simulink model "flythedrone"  (R2019b)
settings: Solver=FixedStepAuto  StartTime=0.0  StopTime=100  RelTol=1e-3
InitFcn:
  | load('BusDefinitions.mat')
values from neighbouring files (symbols this model uses):
  A1_kalman = eval(subs(A1_sampled, t))    [simulation_matlab.m]
  A2_kalman = eval(subs(A2_sampled, t))    [simulation_matlab.m]
  A_s_double = eval(subs(Ad_double,Ts))    [simulation_matlab.m]
  A_s_single = eval(subs(Ad_single,Ts))    [simulation_matlab.m]
  B1_kalman = eval(subs(B1_sampled, t))    [simulation_matlab.m]
  B2_kalman = eval(subs(B2_sampled, t))    [simulation_matlab.m]
  B_s_double = eval(subs(Bd_double,Ts))    [simulation_matlab.m]
  B_s_single = eval(subs(Bd_single,Ts))    [simulation_matlab.m]
  C1_kalman = C1_sampled    [simulation_matlab.m]
  C2_kalman = C2_sampled    [simulation_matlab.m]
  C_double = [1 0]    [simulation_matlab.m]
  C_single = [1]    [simulation_matlab.m]
  D1_kalman = D1_sampled    [simulation_matlab.m]
  D2_kalman = D2_sampled    [simulation_matlab.m]
  D_double = [0]    [simulation_matlab.m]
  D_single = [0]    [simulation_matlab.m]
  Kaileron = lqr(Aaileron, Baileron, Qaileron, Raileron)    [simulation_matlab.m]
  Kelevator = lqr(Aelevator, Belevator, Qelevator, Relevator)    [simulation_matlab.m]
  Krudder = lqr(Arudder, Brudder, Qrudder, Rrudder)    [simulation_matlab.m]
  Kthrust = lqr(Athrust, Bthrust, Qthrust, Rthrust)    [simulation_matlab.m]
  M_motor = [1, 1, 1, -1;             1, 1, -1, 1;             1, -1, -1, -1;             1, -1, 1, 1 ]    [simulation_matlab.m]
  omega_c = 2*pi *20    (= 125.663706144)    [simulation_matlab.m]
  q1_noise = 1    [simulation_matlab.m]
  q2_noise = 1    [simulation_matlab.m]
  q3_noise = 1    [simulation_matlab.m]
  q4_noise = 1    [simulation_matlab.m]
  q5_noise = 1    [simulation_matlab.m]
  q_single = cov(out.In_Out_Data{1}.Values.Data)*10000000000000    [simulation_matlab.m]
  r1_noise = 100    [simulation_matlab.m]
  r2_noise = 100    [simulation_matlab.m]
  r3_noise = 100    [simulation_matlab.m]
  r4_noise = 100    [simulation_matlab.m]
  r5_noise = 100    [simulation_matlab.m]
  r_single = cov(out.In_Out_Data{2}.Values.Data)    [simulation_matlab.m]
  Ts = 0.005    [simulation_matlab.m]
undefined symbols (not defined in the file or in its folder): codertarget, DiscIntNeverNeededParam, Discrete, Time
libraries: ctrlSharedLib x12, simulink x1
settings Model: ExtModeTrigDuration=80  Creator=Sankalp Bhan  LastModifiedBy=cwhipp
settings OptimizationCC: PassReuseOutputArgsThreshold=0  MaxStackSize=64
settings DebuggingCC: ParameterTunabilityLossMsg=error  ArithmeticOperatorsInVariantConditions=warning
settings HardwareCC: ProdBitPerPointer=32  ProdBitPerSizeT=32  ProdBitPerPtrDiffT=32  ProdLargestAtomicInteger=Long  ProdWordSize=32  ProdHWDeviceType=ARM Compatible->ARM 9  UseEmbeddedCoderFeatures=off
settings SFSimCC: SimUseLocalCustomCode=off  MATLABDynamicMemAlloc=off
settings RTWCC: SystemTargetFile=ert.tlc  HardwareBoard=PARROT Mambo  TLCOptions="-aInlineSetEventsForThisBaseRateFcn=TLC_FALSE -aSuppressMultiTaskScheduler=TLC_FALSE   -aRateBasedStepFcn=1"  TemplateMakefile=ert_default_tmf  GenerateReport=on  RTWUseLocalCustomCode=off  Toolchain=Sourcery G++ Lite GNU Toolchain for Drones  LaunchReport=on
settings CodeAppCC: ForceParamTrailComments=on  OperatorAnnotations=on  StateflowObjectComments=on
settings ERTTargetCC: ERTCustomFileBanners=off  MatFileLogging=on  SupportContinuousTime=on  SupportNonInlinedSFcns=on  RemoveResetFunc=off  ModelStepFunctionPrototypeControlCompliant=off

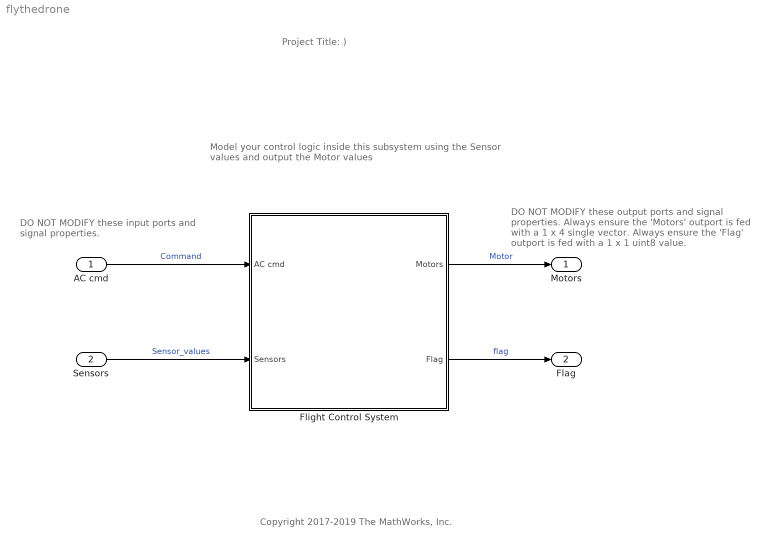
== system flythedrone ==
  note: Model your control logic inside this subsystem
      | using the Sensor values and output the
      | Motor values
  note: DO NOT MODIFY these output ports
      | and signal properties.
      |
      |
      |
      | Always ensure the 'Motors' outport
      | is fed with a 1 x 4 single vector.
      |
      |
      |
      |
      |
      | Always ensure the 'Flag' outport is
      | fed with a 1 x 1 uint8 value.
  note: DO NOT MODIFY these input
      | ports and signal properties.
  note: Copyright 2017-2019 The MathWorks, Inc.
  note: Project Title: )
  AC cmd : Inport  OutDataTypeStr=Bus: CommandBus  BusOutputAsStruct=on
  Sensors : Inport  Port=2  OutDataTypeStr=Bus: SensorsBus  BusOutputAsStruct=on
  Flight Control System : Subsystem  InitFcn=codertarget.parrot.internal.fcsSubsystemCallback(gcb);
  Motors : Outport  OutDataTypeStr=single  PortDimensions=[1 4]  VectorParamsAs1DForOutWhenUnconnected=off
  Flag : Outport  Port=2  OutDataTypeStr=uint8  PortDimensions=1  VectorParamsAs1DForOutWhenUnconnected=off
  wires:
  Flight Control System/1(Motors) -> Motors/1  "Motor"
  AC cmd/1 -> Flight Control System/1(AC cmd)  "Command"
  Sensors/1 -> Flight Control System/2(Sensors)  "Sensor_values"
  Flight Control System/2(Flag) -> Flag/1  "flag"

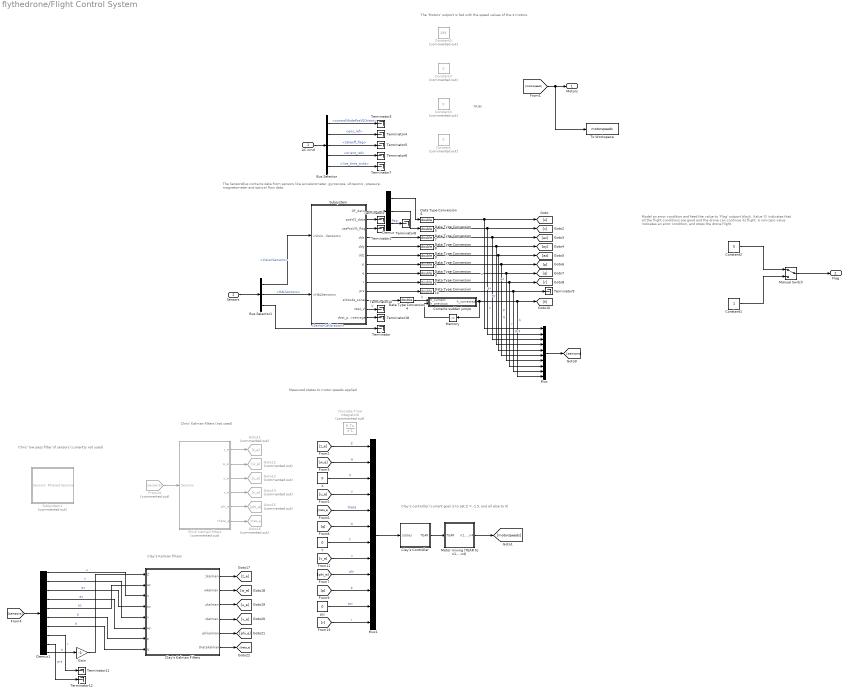
== system flythedrone/Flight Control System ==
  note: Measured states to motor speeds applied
  note: TRIM
  note: The 'Motors' outport is fed with the speed values of the 4 motors.
  note: Model an error condition and feed the value to 'Flag' outport block.
      | Value '0' indicates that all the flight conditions are good and the drone
      | can continue its flight.
      | A non-zero value indicates an error condition, and stops the drone
      | flight.
  note: The SensorsBus contains data from sensors like
      | accelerometer, gyroscope, ultrasonic, pressure,
      | magnetometer and optical flow data.
  note: Chris' Kalman filters (not used)
  note: Chris' low pass filter of sensors
      | (currently not used)
  note: Clay's Kalman filters
  note: Clay's controller (current goal is to set Z = -1.5, and all else to 0)
  AC cmd : Inport
  Sensors : Inport  Port=2
  Bus Selector : BusSelector  OutputSignals=controlModePosVSOrient,pos_ref,takeoff_flag,orient_ref,live_time_ticks
  Bus Selector1 : BusSelector  OutputSignals=VisionSensors,HALSensors,SensorCalibration
  Chris' kalman filters : Subsystem  Commented=on
  Clay's Controller : Subsystem
  Clay's Kalman Filters : Subsystem
  Constant : Constant  Commented=on  Value=0  SampleTime=Ts
  Constant1 : Constant  OutDataTypeStr=uint8
  Constant2 : Constant  Value=0  OutDataTypeStr=uint8
  Constant3 : Constant  Commented=on  Value=0  SampleTime=Ts
  Constant4 : Constant  Commented=on  Value=0  SampleTime=Ts
  Constant5 : Constant  Commented=on  Value=293  SampleTime=Ts
  Corrects sudden jumps : MATLAB Function  TreatAsAtomicUnit=on
  Data Type Conversion{1..10} (10 alike) : DataTypeConversion  OutDataTypeStr=double
  Demux : Demux  Outputs=3
  Demux1 : Demux  Outputs=10
  Discrete-Time Integrator6 : DiscreteIntegrator  Commented=on  SampleTime=-1  ICPrevOutput=DiscIntNeverNeededParam  ICPrevScaledInput=DiscIntNeverNeededParam
  From14 : From  Commented=on  GotoTag=sensors
  Gain : Gain  Gain=-1
  Goto11 : Goto  Commented=on  GotoTag=z_e
  Goto12 : Goto  Commented=on  GotoTag=w_e
  Goto13 : Goto  Commented=on  GotoTag=u_e
  Goto14 : Goto  Commented=on  GotoTag=v_e
  Goto15 : Goto  Commented=on  GotoTag=phi_e
  Goto16 : Goto  Commented=on  GotoTag=theta_e
  Manual Switch : ManualSwitch
  Memory : Memory
  Motor mixing (TEAR to n1,...,n4) : Subsystem
  Mux : Mux  Inputs=10
  Mux1 : Mux  Inputs=12
  Subsystem : Subsystem
  Subsystem1 : Subsystem  Commented=on
  Terminator{,1..12,18} (14 alike) : Terminator
  To Workspace : ToWorkspace  VariableName=motorspeeds  SaveFormat=Structure With Time  SampleTime=-1
  X : Constant  Value=0  SampleTime=0.005
  Y : Constant  Value=0  SampleTime=0.005
  psi : Constant  Value=0  SampleTime=0.005
  Motors : Outport  VectorParamsAs1DForOutWhenUnconnected=off
  Flag : Outport  Port=2  VectorParamsAs1DForOutWhenUnconnected=off
  wires:
  AC cmd/1 -> Bus Selector/1
  Sensors/1 -> Bus Selector1/1
  Bus Selector/1 -> Terminator3/1  "<controlModePosVSOrient>"
  Bus Selector/2 -> Terminator4/1  "<pos_ref>"
  Bus Selector/3 -> Terminator5/1  "<takeoff_flag>"
  Bus Selector/4 -> Terminator6/1  "<orient_ref>"
  Bus Selector/5 -> Terminator7/1  "<live_time_ticks>"
  Manual Switch/1 -> Flag/1
  Constant2/1 -> Manual Switch/1
  Constant1/1 -> Manual Switch/2
  [motorspeeds] -> To Workspace/1, Motors/1
  Bus Selector1/1 -> Subsystem/1(<VisionSensors>)  "<VisionSensors>"
  Bus Selector1/2 -> Subsystem/2(<HALSensors>)  "<HALSensors>"
  Bus Selector1/3 -> Terminator/1  "<SensorCalibration>"
  Subsystem/1(OF_data) -> Demux/1
  Subsystem/4(ddx) -> Data Type Conversion7/1
  Subsystem/5(ddy) -> Data Type Conversion8/1
  Subsystem/6(ddz) -> Data Type Conversion9/1
  Subsystem/7(p) -> Data Type Conversion2/1
  Subsystem/9(r) -> Data Type Conversion1/1
  Subsystem/11(altitude_sonar) -> Data Type Conversion4/1
  Subsystem/13(vbat_percentage) -> Terminator18/1
  Subsystem/8(q) -> Data Type Conversion3/1
  Subsystem/3(usePosVIS_flag) -> Terminator1/1
  Subsystem/2(posVIS_data) -> Terminator2/1
  Demux/1 -> Data Type Conversion6/1
  Demux/2 -> Data Type Conversion5/1
  Demux/3 -> Terminator8/1  "flag"
  Subsystem/10(prs) -> Data Type Conversion10/1
  Data Type Conversion1/1 -> Mux/8, [r]  "r"
  Data Type Conversion2/1 -> Mux/6, [p]  "p"
  Data Type Conversion3/1 -> Mux/7, [q]  "q"
  Data Type Conversion5/1 -> Mux/2, [v]  "v"
  Data Type Conversion6/1 -> [u], Mux/1  "u"
  Data Type Conversion7/1 -> Mux/3, [ax]  "ax"
  Data Type Conversion8/1 -> Mux/4, [ay]  "ay"
  Data Type Conversion9/1 -> Mux/5, [az]  "az"
  Data Type Conversion10/1 -> Mux/9, Terminator9/1  "prs"
  Subsystem/12(vbat_V) -> Terminator10/1  "V"
  Mux1/1 -> Clay's Controller/1(states)
  Motor mixing (TEAR to n1,...,n4)/1(n1,...,n4) -> [motorspeeds]
  [z_e] -> Mux1/1  "Z"
  [w_e] -> Mux1/2  "w"
  [u_e] -> Mux1/4  "u"
  [theta_e] -> Mux1/5  "theta"
  [q] -> Mux1/6  "q"
  Y/1 -> Mux1/7  "Y"
  [p] -> Mux1/10  "p"
  [phi_e] -> Mux1/9  "phi"
  [v_e] -> Mux1/8  "v"
  psi/1 -> Mux1/11  "psi"
  [r] -> Mux1/12  "r"
  Clay's Controller/1(TEAR) -> Motor mixing (TEAR to n1,...,n4)/1(TEAR)
  Mux/1 -> [sensors]
  From14/1 -> Chris' kalman filters/1(Sensors)
  Chris' kalman filters/1(z_e) -> Goto11/1
  Chris' kalman filters/2(w_e) -> Goto12/1
  Chris' kalman filters/3(u_e) -> Goto13/1
  Chris' kalman filters/4(v_e) -> Goto14/1
  Chris' kalman filters/5(phi_e) -> Goto15/1
  Chris' kalman filters/6(theta_e) -> Goto16/1
  X/1 -> Mux1/3  "X"
  Data Type Conversion4/1 -> Corrects sudden jumps/1(h_current)  "h"
  Corrects sudden jumps/1(h_corrected) -> [h], Mux/10, Memory/1  "h"
  Memory/1 -> Corrects sudden jumps/2(h_previous)
  Clay's Kalman Filters/6(thetakalman) -> [theta_e]
  Clay's Kalman Filters/1(zkalman) -> [z_e]
  Clay's Kalman Filters/5(phikalman) -> [phi_e]
  Clay's Kalman Filters/2(wkalman) -> [w_e]
  Clay's Kalman Filters/3(ukalman) -> [u_e]
  Clay's Kalman Filters/4(vkalman) -> [v_e]
  [sensors] -> Demux1/1
  Demux1/1 -> Clay's Kalman Filters/3(u)  "u"
  Demux1/2 -> Clay's Kalman Filters/5(v)  "v"
  Demux1/3 -> Clay's Kalman Filters/4(ax)  "ax"
  Demux1/4 -> Clay's Kalman Filters/6(ay)  "ay"
  Demux1/5 -> Clay's Kalman Filters/2(az)  "az"
  Demux1/6 -> Clay's Kalman Filters/7(p)  "p"
  Demux1/7 -> Clay's Kalman Filters/8(q)  "q"
  Demux1/8 -> Terminator11/1  "r"
  Gain/1 -> Clay's Kalman Filters/1(Z)
  Demux1/10 -> Gain/1  "h"
  Demux1/9 -> Terminator12/1  "prs"

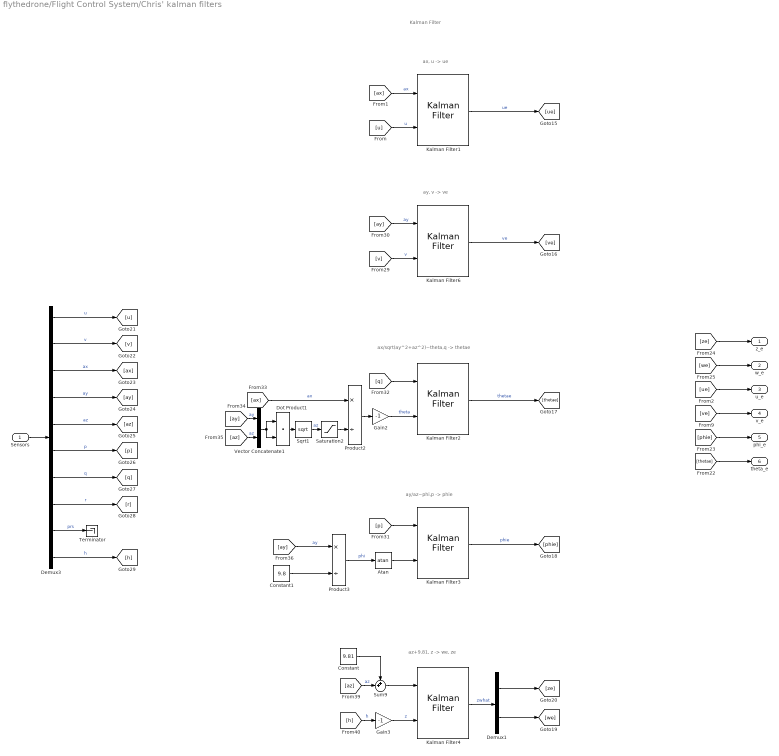
== system flythedrone/Flight Control System/Chris' kalman filters ==
  note: Kalman Filter
  note: ay, v -> ve
  note: ax, u -> ue
  note: ax/sqrt(ay^2+az^2)~theta,q -> thetae
  note: ay/az~phi,p -> phie
  note: az+9.81, z -> we, ze
  Sensors : Inport
  Atan : Trigonometry  Operator=atan
  Constant : Constant  Value=9.81
  Constant1 : Constant  Value=9.8
  Demux1 : Demux  Outputs=2
  Demux3 : Demux  Outputs=10
  Dot Product1 : DotProduct  OutMin=0.0001  InputSameDT=on  OutDataTypeStr=Inherit: Inherit via internal rule
  Gain2 : Gain  Gain=-1
  Gain3 : Gain  Gain=-1
  Kalman Filter{1..3,6} (4 alike) : ctrlSharedLib/Kalman Filter  TimeDomain=Discrete-Time  UseCurrentEstimator=on  ModelSource=Individual A, B, C, D matrices  ModelSourceVariable=ss(0.95,1,1,0,1)  A=A_s_single  B=B_s_single  C=C_single  D=D_single  NumberOfStates=1  NumberOfInputs=1  NumberOfOutputs=1  InitialEstimateSource=Dialog  X0=[0]  P0=10  UseK=off  UseGH=off  NumberOfProcessNoiseInputs=1  G=1  TimeInvariantG=on  H=0  TimeInvariantH=on  Q=[1]*q_single  TimeInvariantQ=on  R=[1]*r_single*10000  TimeInvariantR=on  N=0  TimeInvariantN=on  AddInputPort=on  AddEnablePort=off  OutputEstimatedY=off  OutputP=off  Ts=Ts
      settings: SourceProductBaseCode=CT
  Kalman Filter4 : ctrlSharedLib/Kalman Filter  TimeDomain=Discrete-Time  UseCurrentEstimator=on  ModelSource=Individual A, B, C, D matrices  ModelSourceVariable=ss(0.95,1,1,0,1)  A=A_s_double  B=B_s_double  C=C_double  D=D_double  NumberOfStates=1  NumberOfInputs=1  NumberOfOutputs=1  InitialEstimateSource=Dialog  X0=[0]  P0=10  UseK=off  UseGH=off  NumberOfProcessNoiseInputs=1  G=1  TimeInvariantG=on  H=0  TimeInvariantH=on  Q=[0 0; 0 1]*q_single  TimeInvariantQ=on  R=[1]*r_single*10000  TimeInvariantR=on  N=0  TimeInvariantN=on  AddInputPort=on  AddEnablePort=off  OutputEstimatedY=off  OutputP=off  Ts=Ts
      settings: SourceProductBaseCode=CT
  Product2 : Product  Inputs=*/
  Product3 : Product  Inputs=*/
  Saturation2 : Saturate  UpperLimit=inf  LowerLimit=0.001
  Sqrt1 : Sqrt  SaturateOnIntegerOverflow=on
  Sum9 : Sum  Inputs=++|
  Terminator : Terminator
  Vector Concatenate1 : Concatenate
  z_e : Outport
  w_e : Outport  Port=2
  u_e : Outport  Port=3
  v_e : Outport  Port=4
  phi_e : Outport  Port=5
  theta_e : Outport  Port=6
  wires:
  [h] -> Gain3/1  "h"
  Kalman Filter1/1 -> [ue]  "ue"
  Kalman Filter6/1 -> [ve]  "ve"
  Kalman Filter2/1 -> [thetae]  "thetae"
  Kalman Filter3/1 -> [phie]  "phie"
  Demux1/2 -> [we]
  Demux1/1 -> [ze]
  Gain3/1 -> Kalman Filter4/2  "z"
  Kalman Filter4/1 -> Demux1/1  "zwhat"
  [ay] -> Product3/1  "ay"
  Product3/1 -> Atan/1  "phi"
  [p] -> Kalman Filter3/1
  [ay] -> Vector Concatenate1/1  "ay"
  [az] -> Vector Concatenate1/2  "az"
  Vector Concatenate1/1 -> Dot Product1/1, Dot Product1/2
  Dot Product1/1 -> Sqrt1/1
  [ax] -> Product2/1  "ax"
  Product2/1 -> Gain2/1
  Sqrt1/1 -> Saturation2/1  "az"
  Saturation2/1 -> Product2/2
  Gain2/1 -> Kalman Filter2/2  "theta"
  [q] -> Kalman Filter2/1
  [ay] -> Kalman Filter6/1  "ay"
  [v] -> Kalman Filter6/2  "v"
  [u] -> Kalman Filter1/2  "u"
  [ax] -> Kalman Filter1/1  "ax"
  [az] -> Sum9/2  "az"
  Sum9/1 -> Kalman Filter4/1
  Constant/1 -> Sum9/1
  Demux3/1 -> [u]  "u"
  Sensors/1 -> Demux3/1
  Demux3/6 -> [p]  "p"
  Atan/1 -> Kalman Filter3/2
  Constant1/1 -> Product3/2
  [ze] -> z_e/1
  [we] -> w_e/1
  [ve] -> v_e/1
  [ue] -> u_e/1
  [phie] -> phi_e/1
  [thetae] -> theta_e/1
  Demux3/3 -> [ax]  "ax"
  Demux3/2 -> [v]  "v"
  Demux3/7 -> [q]  "q"
  Demux3/4 -> [ay]  "ay"
  Demux3/5 -> [az]  "az"
  Demux3/10 -> [h]  "h"
  Demux3/8 -> [r]  "r"
  Demux3/9 -> Terminator/1  "prs"

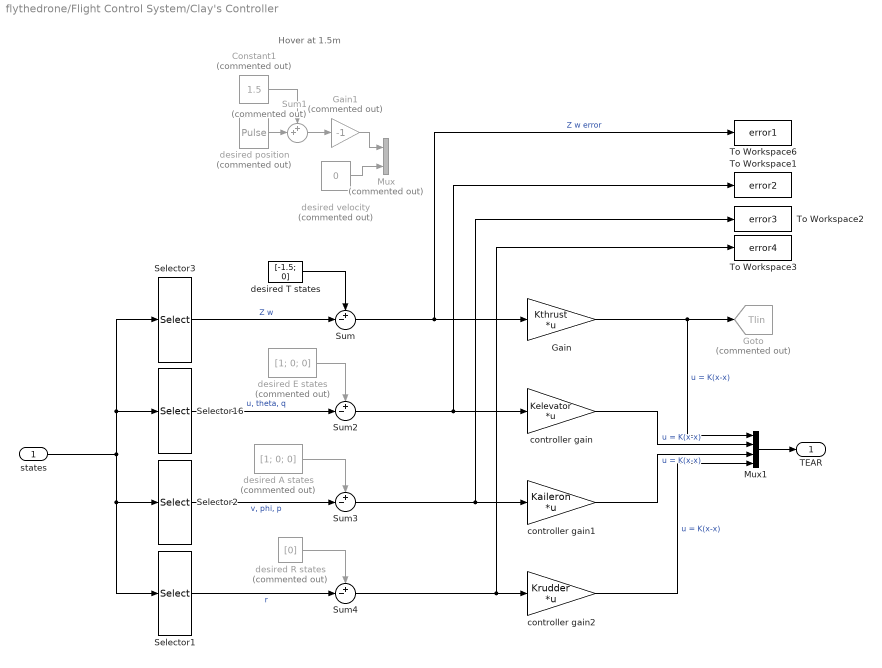
== system flythedrone/Flight Control System/Clay's Controller ==
  note: Hover at 1.5m
  states : Inport
  Constant1 : Constant  Commented=on  Value=1.5  SampleTime=0.05
  Gain : Gain  Gain=Kthrust  Multiplication=Matrix(K*u)
  Gain1 : Gain  Commented=on  Gain=-1
  Goto : Goto  Commented=on  GotoTag=Tlin  TagVisibility=global
  Mux : Mux  Commented=on  Inputs=2
  Mux1 : Mux
  Selector1 : Selector  InputPortWidth=12  IndexOptions=Index vector (dialog)  Indices=[12]  OutputSizes=1
  Selector16 : Selector  InputPortWidth=12  IndexOptions=Index vector (dialog)  Indices=[4 5 6]  OutputSizes=1
  Selector2 : Selector  InputPortWidth=12  IndexOptions=Index vector (dialog)  Indices=[8 9 10]  OutputSizes=1
  Selector3 : Selector  InputPortWidth=12  IndexOptions=Index vector (dialog)  Indices=[1 2]  OutputSizes=1
  Sum{,2..4} (4 alike) : Sum  Inputs=+-|
  Sum1 : Sum  Commented=on  Inputs=++|
  To Workspace1 : ToWorkspace  VariableName=error2  SaveFormat=Structure With Time  SampleTime=-1
  To Workspace2 : ToWorkspace  VariableName=error3  SaveFormat=Structure With Time  SampleTime=-1
  To Workspace3 : ToWorkspace  VariableName=error4  SaveFormat=Structure With Time  SampleTime=-1
  To Workspace6 : ToWorkspace  VariableName=error1  SaveFormat=Structure With Time  SampleTime=-1
  controller gain : Gain  Gain=Kelevator  Multiplication=Matrix(K*u)
  controller gain1 : Gain  Gain=Kaileron  Multiplication=Matrix(K*u)
  controller gain2 : Gain  Gain=Krudder  Multiplication=Matrix(K*u)
  desired A states : Constant  Commented=on  Value=[1; 0; 0]  SampleTime=0.005
  desired E states : Constant  Commented=on  Value=[1; 0; 0]  SampleTime=0.005
  desired R states : Constant  Commented=on  Value=[0]  SampleTime=0.005
  desired T states : Constant  Value=[-1.5; 0]  SampleTime=0.005
  desired position : DiscretePulseGenerator  Commented=on  PulseType=Time based  Amplitude=-1.5  Period=10  PulseWidth=50
  desired velocity : Constant  Commented=on  Value=0  SampleTime=0.05
  TEAR : Outport
  wires:
  states/1 -> Selector16/1, Selector3/1, Selector2/1, Selector1/1
  desired T states/1 -> Sum/1
  Sum/1 -> To Workspace6/1, Gain/1  "Z w error"
  Gain/1 -> Goto/1, Mux1/1  "u = K(x-x)"
  desired E states/1 -> Sum2/1
  Sum2/1 -> To Workspace1/1, controller gain/1
  controller gain/1 -> Mux1/2  "u = K(x-x)"
  controller gain1/1 -> Mux1/3  "u = K(x-x)"
  desired A states/1 -> Sum3/1
  controller gain2/1 -> Mux1/4  "u = K(x-x)"
  Sum4/1 -> To Workspace3/1, controller gain2/1
  desired R states/1 -> Sum4/1
  Selector3/1 -> Sum/2  "Z w"
  Selector16/1 -> Sum2/2  "u, theta, q"
  Selector2/1 -> Sum3/2  "v, phi, p"
  Selector1/1 -> Sum4/2  "r"
  Mux1/1 -> TEAR/1
  Sum1/1 -> Gain1/1
  desired position/1 -> Sum1/2
  Gain1/1 -> Mux/1
  desired velocity/1 -> Mux/2
  Constant1/1 -> Sum1/1
  Sum3/1 -> To Workspace2/1, controller gain1/1

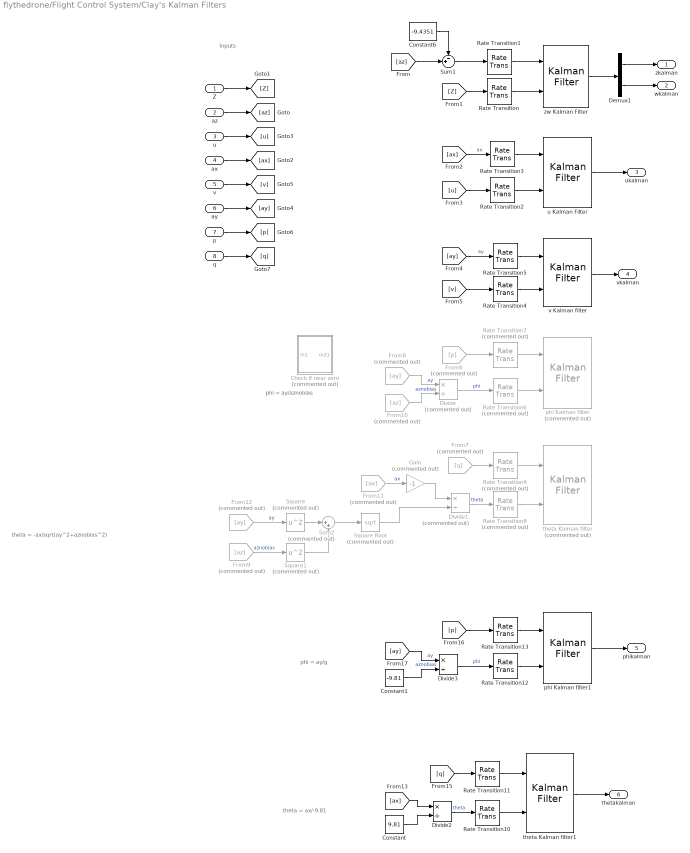
== system flythedrone/Flight Control System/Clay's Kalman Filters ==
  note: Inputs
  note: phi = ay/aznobias
  note: theta = -ax/sqrt(ay^2+aznobias^2)
  note: theta = ax/-9.81
  note: phi = ay/g
  Z : Inport
  az : Inport  Port=2
  u : Inport  Port=3
  ax : Inport  Port=4
  v : Inport  Port=5
  ay : Inport  Port=6
  p : Inport  Port=7
  q : Inport  Port=8
  Check if near zero : Subsystem  Commented=on
  Constant : Constant  Value=9.81  SampleTime=0.005
  Constant1 : Constant  Value=-9.81  SampleTime=0.005
  Constant6 : Constant  Value=-9.4351
  Demux1 : Demux  Outputs=2
  Divide : Product  Commented=on  Inputs=*/
  Divide1 : Product  Commented=on  Inputs=*/
  Divide2 : Product  Inputs=*/
  Divide3 : Product  Inputs=*/
  From10 : From  Commented=on  GotoTag=az
  From11 : From  Commented=on  GotoTag=ax
  From12 : From  Commented=on  GotoTag=ay
  From6 : From  Commented=on  GotoTag=p
  From7 : From  Commented=on  GotoTag=q
  From8 : From  Commented=on  GotoTag=ay
  From9 : From  Commented=on  GotoTag=az
  Gain : Gain  Commented=on  Gain=-1
  Rate Transition{,1..5,10..13} (10 alike) : RateTransition  OutPortSampleTime=0.005
  Rate Transition{6..9} (4 alike) : RateTransition  Commented=on  OutPortSampleTime=0.005
  Square : Math  Commented=on  Operator=square  SignedPower=off  SaturateOnIntegerOverflow=on
  Square Root : Sqrt  Commented=on  SaturateOnIntegerOverflow=on
  Square1 : Math  Commented=on  Operator=square  SignedPower=off  SaturateOnIntegerOverflow=on
  Sum1 : Sum  Inputs=-+|
  Sum2 : Sum  Commented=on  Inputs=|++
  phi Kalman filter : ctrlSharedLib/Kalman Filter  Commented=on  TimeDomain=Discrete-Time  UseCurrentEstimator=on  ModelSource=Individual A, B, C, D matrices  ModelSourceVariable=ss(0.95,1,1,0,1)  A=A2_kalman  B=B2_kalman  C=C2_kalman  D=D2_kalman  NumberOfStates=1  NumberOfInputs=1  NumberOfOutputs=1  InitialEstimateSource=Dialog  X0=[0]  P0=10  UseK=off  UseGH=off  NumberOfProcessNoiseInputs=1  G=1  TimeInvariantG=on  H=0  TimeInvariantH=on  Q=q4_noise;  TimeInvariantQ=on  R=r4_noise;  TimeInvariantR=on  N=0  TimeInvariantN=on  AddInputPort=on  AddEnablePort=off  OutputEstimatedY=off  OutputP=off  Ts=-1
      settings: SourceProductBaseCode=CT
  phi Kalman filter1 : ctrlSharedLib/Kalman Filter  TimeDomain=Discrete-Time  UseCurrentEstimator=on  ModelSource=Individual A, B, C, D matrices  ModelSourceVariable=ss(0.95,1,1,0,1)  A=A2_kalman  B=B2_kalman  C=C2_kalman  D=D2_kalman  NumberOfStates=1  NumberOfInputs=1  NumberOfOutputs=1  InitialEstimateSource=Dialog  X0=[0]  P0=10  UseK=off  UseGH=off  NumberOfProcessNoiseInputs=1  G=1  TimeInvariantG=on  H=0  TimeInvariantH=on  Q=q4_noise;  TimeInvariantQ=on  R=r4_noise;  TimeInvariantR=on  N=0  TimeInvariantN=on  AddInputPort=on  AddEnablePort=off  OutputEstimatedY=off  OutputP=off  Ts=-1
      settings: SourceProductBaseCode=CT
  theta Kalman filter : ctrlSharedLib/Kalman Filter  Commented=on  TimeDomain=Discrete-Time  UseCurrentEstimator=on  ModelSource=Individual A, B, C, D matrices  ModelSourceVariable=ss(0.95,1,1,0,1)  A=A2_kalman  B=B2_kalman  C=C2_kalman  D=D2_kalman  NumberOfStates=1  NumberOfInputs=1  NumberOfOutputs=1  InitialEstimateSource=Dialog  X0=[0]  P0=10  UseK=off  UseGH=off  NumberOfProcessNoiseInputs=1  G=1  TimeInvariantG=on  H=0  TimeInvariantH=on  Q=q5_noise;  TimeInvariantQ=on  R=r5_noise;  TimeInvariantR=on  N=0  TimeInvariantN=on  AddInputPort=on  AddEnablePort=off  OutputEstimatedY=off  OutputP=off  Ts=-1
      settings: SourceProductBaseCode=CT
  theta Kalman filter1 : ctrlSharedLib/Kalman Filter  TimeDomain=Discrete-Time  UseCurrentEstimator=on  ModelSource=Individual A, B, C, D matrices  ModelSourceVariable=ss(0.95,1,1,0,1)  A=A2_kalman  B=B2_kalman  C=C2_kalman  D=D2_kalman  NumberOfStates=1  NumberOfInputs=1  NumberOfOutputs=1  InitialEstimateSource=Dialog  X0=[0]  P0=10  UseK=off  UseGH=off  NumberOfProcessNoiseInputs=1  G=1  TimeInvariantG=on  H=0  TimeInvariantH=on  Q=q5_noise;  TimeInvariantQ=on  R=r5_noise;  TimeInvariantR=on  N=0  TimeInvariantN=on  AddInputPort=on  AddEnablePort=off  OutputEstimatedY=off  OutputP=off  Ts=-1
      settings: SourceProductBaseCode=CT
  u Kalman Filter : ctrlSharedLib/Kalman Filter  TimeDomain=Discrete-Time  UseCurrentEstimator=on  ModelSource=Individual A, B, C, D matrices  ModelSourceVariable=ss(0.95,1,1,0,1)  A=A2_kalman  B=B2_kalman  C=C2_kalman  D=D2_kalman  NumberOfStates=1  NumberOfInputs=1  NumberOfOutputs=1  InitialEstimateSource=Dialog  X0=[0]  P0=10  UseK=off  UseGH=off  NumberOfProcessNoiseInputs=1  G=1  TimeInvariantG=on  H=0  TimeInvariantH=on  Q=q2_noise;  TimeInvariantQ=on  R=r2_noise;  TimeInvariantR=on  N=0  TimeInvariantN=on  AddInputPort=on  AddEnablePort=off  OutputEstimatedY=off  OutputP=off  Ts=-1
      settings: SourceProductBaseCode=CT
  v Kalman filter : ctrlSharedLib/Kalman Filter  TimeDomain=Discrete-Time  UseCurrentEstimator=on  ModelSource=Individual A, B, C, D matrices  ModelSourceVariable=ss(0.95,1,1,0,1)  A=A2_kalman  B=B2_kalman  C=C2_kalman  D=D2_kalman  NumberOfStates=1  NumberOfInputs=1  NumberOfOutputs=1  InitialEstimateSource=Dialog  X0=[0]  P0=10  UseK=off  UseGH=off  NumberOfProcessNoiseInputs=1  G=1  TimeInvariantG=on  H=0  TimeInvariantH=on  Q=q3_noise;  TimeInvariantQ=on  R=r3_noise;  TimeInvariantR=on  N=0  TimeInvariantN=on  AddInputPort=on  AddEnablePort=off  OutputEstimatedY=off  OutputP=off  Ts=-1
      settings: SourceProductBaseCode=CT
  zw Kalman Filter : ctrlSharedLib/Kalman Filter  TimeDomain=Discrete-Time  UseCurrentEstimator=on  ModelSource=Individual A, B, C, D matrices  ModelSourceVariable=ss(0.95,1,1,0,1)  A=A1_kalman  B=B1_kalman  C=C1_kalman  D=D1_kalman  NumberOfStates=1  NumberOfInputs=1  NumberOfOutputs=1  InitialEstimateSource=Dialog  X0=[0;0 ]  P0=10  UseK=off  UseGH=off  NumberOfProcessNoiseInputs=1  G=1  TimeInvariantG=on  H=0  TimeInvariantH=on  Q=[0 0 ; 0 1].*q1_noise;  TimeInvariantQ=on  R=r1_noise;  TimeInvariantR=on  N=0  TimeInvariantN=on  AddInputPort=on  AddEnablePort=off  OutputEstimatedY=off  OutputP=off  Ts=-1
      settings: SourceProductBaseCode=CT
  zkalman : Outport
  wkalman : Outport  Port=2
  ukalman : Outport  Port=3
  vkalman : Outport  Port=4
  phikalman : Outport  Port=5
  thetakalman : Outport  Port=6
  wires:
  zw Kalman Filter/1 -> Demux1/1
  Divide1/1 -> Rate Transition8/1  "theta"
  Rate Transition6/1 -> phi Kalman filter/2
  From6/1 -> Rate Transition7/1
  Square/1 -> Sum2/1
  Rate Transition/1 -> zw Kalman Filter/2
  [v] -> Rate Transition4/1
  Demux1/2 -> wkalman/1
  Rate Transition1/1 -> zw Kalman Filter/1
  Rate Transition3/1 -> u Kalman Filter/1
  From7/1 -> Rate Transition9/1
  Rate Transition4/1 -> v Kalman filter/2
  Gain/1 -> Divide1/1
  From9/1 -> Square1/1  "aznobias"
  [ax] -> Rate Transition3/1  "ax"
  Rate Transition7/1 -> phi Kalman filter/1
  Rate Transition5/1 -> v Kalman filter/1
  Divide/1 -> Rate Transition6/1  "phi"
  u Kalman Filter/1 -> ukalman/1
  Sum2/1 -> Square Root/1
  [u] -> Rate Transition2/1
  Rate Transition2/1 -> u Kalman Filter/2
  [Z] -> Rate Transition/1
  Rate Transition9/1 -> theta Kalman filter/1
  Square Root/1 -> Divide1/2
  Square1/1 -> Sum2/2
  Demux1/1 -> zkalman/1
  v Kalman filter/1 -> vkalman/1
  [ay] -> Rate Transition5/1  "ay"
  Rate Transition8/1 -> theta Kalman filter/2
  [az] -> Sum1/2
  Constant6/1 -> Sum1/1
  Sum1/1 -> Rate Transition1/1
  az/1 -> [az]
  ax/1 -> [ax]
  ay/1 -> [ay]
  v/1 -> [v]
  p/1 -> [p]
  q/1 -> [q]
  From8/1 -> Divide/1  "ay"
  From10/1 -> Divide/2  "aznobias"
  From11/1 -> Gain/1  "ax"
  From12/1 -> Square/1  "ay"
  Z/1 -> [Z]
  u/1 -> [u]
  [ax] -> Divide2/1
  Rate Transition10/1 -> theta Kalman filter1/2
  Rate Transition11/1 -> theta Kalman filter1/1
  Constant/1 -> Divide2/2
  theta Kalman filter1/1 -> thetakalman/1
  [q] -> Rate Transition11/1
  Divide2/1 -> Rate Transition10/1  "theta"
  Divide3/1 -> Rate Transition12/1  "phi"
  [ay] -> Divide3/1  "ay"
  [p] -> Rate Transition13/1
  Rate Transition12/1 -> phi Kalman filter1/2
  phi Kalman filter1/1 -> phikalman/1
  Rate Transition13/1 -> phi Kalman filter1/1
  Constant1/1 -> Divide3/2  "aznobias"

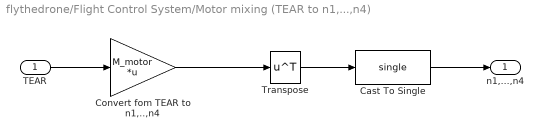
== system flythedrone/Flight Control System/Motor mixing (TEAR to n1,...,n4) ==
  TEAR : Inport
  Cast To Single : DataTypeConversion  OutDataTypeStr=single
  Convert fom TEAR to n1,..,n4 : Gain  Gain=M_motor  Multiplication=Matrix(K*u)
  Transpose : Math  Operator=transpose  SignedPower=off  SaturateOnIntegerOverflow=on
  n1,...,n4 : Outport
  wires:
  TEAR/1 -> Convert fom TEAR to n1,..,n4/1
  Convert fom TEAR to n1,..,n4/1 -> Transpose/1
  Transpose/1 -> Cast To Single/1
  Cast To Single/1 -> n1,...,n4/1

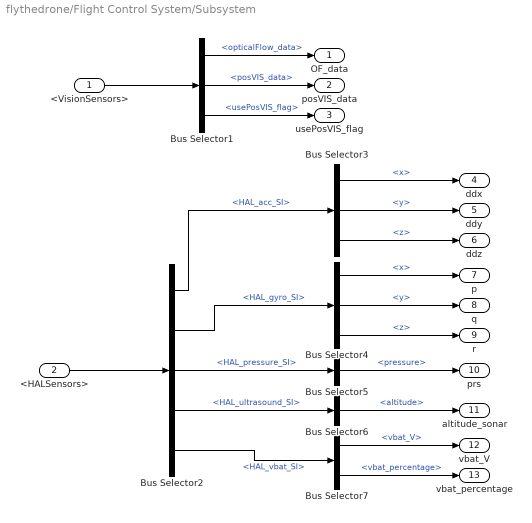
== system flythedrone/Flight Control System/Subsystem ==
  <VisionSensors> : Inport
  <HALSensors> : Inport  Port=2
  Bus Selector1 : BusSelector  OutputSignals=opticalFlow_data,posVIS_data,usePosVIS_flag
  Bus Selector2 : BusSelector  OutputSignals=HAL_acc_SI,HAL_gyro_SI,HAL_pressure_SI,HAL_ultrasound_SI,HAL_vbat_SI
  Bus Selector3 : BusSelector  OutputSignals=x,y,z
  Bus Selector4 : BusSelector  OutputSignals=x,y,z
  Bus Selector5 : BusSelector  OutputSignals=pressure
  Bus Selector6 : BusSelector  OutputSignals=altitude
  Bus Selector7 : BusSelector  OutputSignals=vbat_V,vbat_percentage
  OF_data : Outport  VectorParamsAs1DForOutWhenUnconnected=off
  posVIS_data : Outport  Port=2  VectorParamsAs1DForOutWhenUnconnected=off
  usePosVIS_flag : Outport  Port=3  VectorParamsAs1DForOutWhenUnconnected=off
  ddx : Outport  Port=4  VectorParamsAs1DForOutWhenUnconnected=off
  ddy : Outport  Port=5  VectorParamsAs1DForOutWhenUnconnected=off
  ddz : Outport  Port=6  VectorParamsAs1DForOutWhenUnconnected=off
  p : Outport  Port=7  VectorParamsAs1DForOutWhenUnconnected=off
  q : Outport  Port=8  VectorParamsAs1DForOutWhenUnconnected=off
  r : Outport  Port=9  VectorParamsAs1DForOutWhenUnconnected=off
  prs : Outport  Port=10  VectorParamsAs1DForOutWhenUnconnected=off
  altitude_sonar : Outport  Port=11  VectorParamsAs1DForOutWhenUnconnected=off
  vbat_V : Outport  Port=12  VectorParamsAs1DForOutWhenUnconnected=off
  vbat_percentage : Outport  Port=13  VectorParamsAs1DForOutWhenUnconnected=off
  wires:
  <VisionSensors>/1 -> Bus Selector1/1
  <HALSensors>/1 -> Bus Selector2/1
  Bus Selector1/1 -> OF_data/1  "<opticalFlow_data>"
  Bus Selector1/2 -> posVIS_data/1  "<posVIS_data>"
  Bus Selector1/3 -> usePosVIS_flag/1  "<usePosVIS_flag>"
  Bus Selector2/1 -> Bus Selector3/1  "<HAL_acc_SI>"
  Bus Selector2/2 -> Bus Selector4/1  "<HAL_gyro_SI>"
  Bus Selector2/3 -> Bus Selector5/1  "<HAL_pressure_SI>"
  Bus Selector2/4 -> Bus Selector6/1  "<HAL_ultrasound_SI>"
  Bus Selector2/5 -> Bus Selector7/1  "<HAL_vbat_SI>"
  Bus Selector3/1 -> ddx/1  "<x>"
  Bus Selector3/2 -> ddy/1  "<y>"
  Bus Selector3/3 -> ddz/1  "<z>"
  Bus Selector4/2 -> q/1  "<y>"
  Bus Selector4/1 -> p/1  "<x>"
  Bus Selector4/3 -> r/1  "<z>"
  Bus Selector5/1 -> prs/1  "<pressure>"
  Bus Selector6/1 -> altitude_sonar/1  "<altitude>"
  Bus Selector7/1 -> vbat_V/1  "<vbat_V>"
  Bus Selector7/2 -> vbat_percentage/1  "<vbat_percentage>"

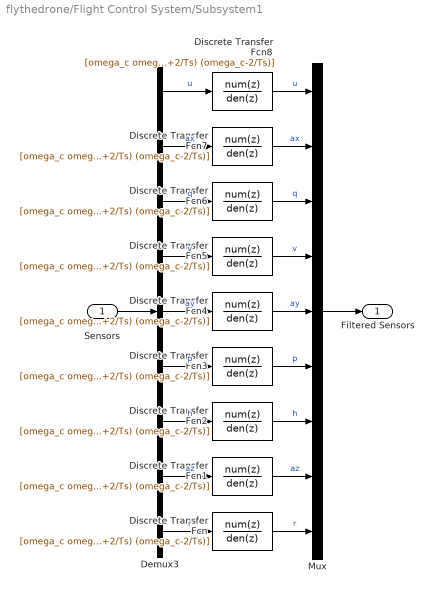
== system flythedrone/Flight Control System/Subsystem1 ==
  Sensors : Inport
  Demux3 : Demux  Outputs=9
  Discrete Transfer Fcn{,2..8} (8 alike) : DiscreteTransferFcn  Numerator=[omega_c omega_c]  Denominator=[(omega_c+2/Ts) (omega_c-2/Ts)]  SampleTime=0.005
  Discrete Transfer Fcn1 : DiscreteTransferFcn  Numerator=[omega_c omega_c]  Denominator=[(omega_c+2/Ts) (omega_c-2/Ts)]  InitialStates=.01  SampleTime=0.005
  Mux : Mux  Inputs=9
  Filtered Sensors : Outport
  wires:
  Demux3/6 -> Discrete Transfer Fcn3/1  "p"
  Demux3/5 -> Discrete Transfer Fcn4/1  "ay"
  Demux3/7 -> Discrete Transfer Fcn2/1  "h"
  Demux3/4 -> Discrete Transfer Fcn5/1  "v"
  Demux3/9 -> Discrete Transfer Fcn/1  "r"
  Demux3/8 -> Discrete Transfer Fcn1/1  "az"
  Demux3/2 -> Discrete Transfer Fcn7/1  "ax"
  Sensors/1 -> Demux3/1
  Demux3/3 -> Discrete Transfer Fcn6/1  "q"
  Demux3/1 -> Discrete Transfer Fcn8/1  "u"
  Discrete Transfer Fcn/1 -> Mux/9  "r"
  Discrete Transfer Fcn1/1 -> Mux/8  "az"
  Discrete Transfer Fcn2/1 -> Mux/7  "h"
  Discrete Transfer Fcn3/1 -> Mux/6  "p"
  Discrete Transfer Fcn4/1 -> Mux/5  "ay"
  Discrete Transfer Fcn5/1 -> Mux/4  "v"
  Discrete Transfer Fcn6/1 -> Mux/3  "q"
  Discrete Transfer Fcn7/1 -> Mux/2  "ax"
  Discrete Transfer Fcn8/1 -> Mux/1  "u"
  Mux/1 -> Filtered Sensors/1

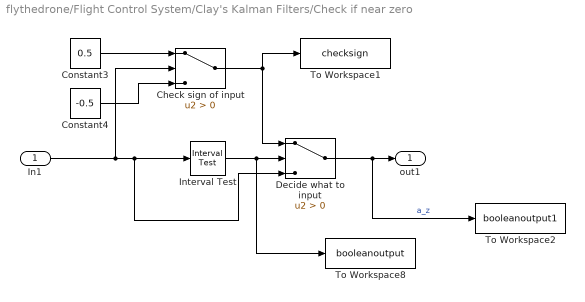
== system flythedrone/Flight Control System/Clay's Kalman Filters/Check if near zero ==
  In1 : Inport
  Check sign of input : Switch  Criteria=u2 > Threshold
  Constant3 : Constant  Value=0.5  SampleTime=0.005
  Constant4 : Constant  Value=-0.5  SampleTime=0.005
  Decide what to input : Switch  Criteria=u2 > Threshold
  Interval Test : simulink/Logic and Bit Operations/Interval Test  IntervalClosedRight=on  uplimit=0.5  IntervalClosedLeft=on  lowlimit=-0.5  OutDataTypeStr=boolean
  To Workspace1 : ToWorkspace  VariableName=checksign  SaveFormat=Structure With Time  SampleTime=-1
  To Workspace2 : ToWorkspace  VariableName=booleanoutput1  SaveFormat=Structure With Time  SampleTime=-1
  To Workspace8 : ToWorkspace  VariableName=booleanoutput  SaveFormat=Structure With Time  SampleTime=-1
  out1 : Outport
  wires:
  Decide what to input/1 -> To Workspace2/1, out1/1  "a_z"
  Interval Test/1 -> To Workspace8/1, Decide what to input/2
  Check sign of input/1 -> Decide what to input/1, To Workspace1/1
  In1/1 -> Check sign of input/2, Interval Test/1, Decide what to input/3
  Constant4/1 -> Check sign of input/3
  Constant3/1 -> Check sign of input/1

== matlab function flythedrone/Flight Control System/Corrects sudden jumps ==
  data: h_current input; h_corrected output; h_previous input
function h_corrected = fcn(h_current, h_previous)

h_change = abs(h_current-h_previous);

diffthreshold = 1;

if(h_change > diffthreshold)
    h_corrected = h_previous;
else
    h_corrected = h_current;
end
